simulink model "foc"  (R2026a)
settings: Solver=VariableStepAuto  FixedStep=5e-5
libraries: mcbcontrolslib x1, mcbplantlib x1, autolibpmsmexterior x1
settings Model: Creator=probst  LastModifiedBy=probst

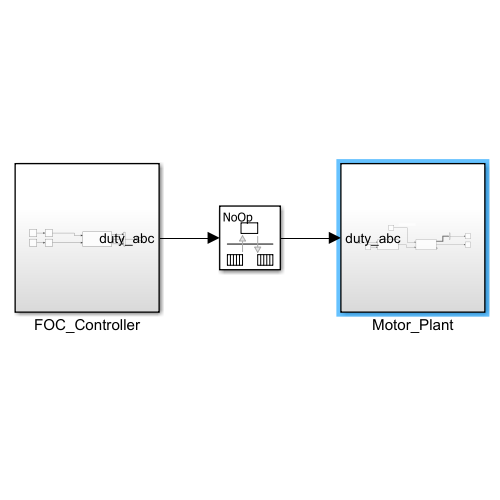
[thumbnail: Simulink's stored preview of the top-level diagram]
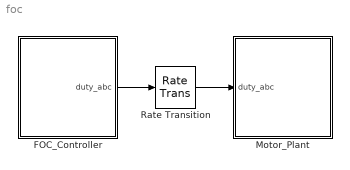
== system foc ==
  FOC_Controller : Subsystem
  Motor_Plant : Subsystem
  Rate Transition : RateTransition
  wires:
  FOC_Controller/1(duty_abc) -> Rate Transition/1
  Rate Transition/1 -> Motor_Plant/1(duty_abc)

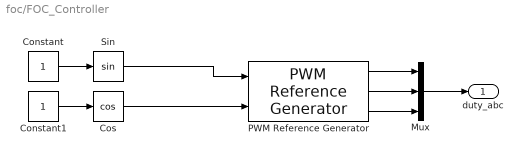
== system foc/FOC_Controller ==
  Constant : Constant
  Constant1 : Constant
  Cos : Trigonometry  Operator=cos
  Mux : Mux  Inputs=3
  PWM Reference Generator : mcbcontrolslib/PWM Reference Generator  modType=SVM: space vector modulation  inSignal=Valphabeta  expandVoltageInput=on  inputUnits=Per-unit  LimitModulation=off  enableVoltage=on  enableModulationSignal=off  enableDutyCycle=off  expandVoltageOutput=on
      settings: LibrarySourceBlock=mcblib/Controls/Math Transforms/PWM Reference Generator
  Sin : Trigonometry  OutputSignalType=real
  duty_abc : Outport
  wires:
  PWM Reference Generator/2 -> Mux/2
  PWM Reference Generator/1 -> Mux/1
  PWM Reference Generator/3 -> Mux/3
  Mux/1 -> duty_abc/1
  Sin/1 -> PWM Reference Generator/1
  Cos/1 -> PWM Reference Generator/2
  Constant/1 -> Sin/1
  Constant1/1 -> Cos/1

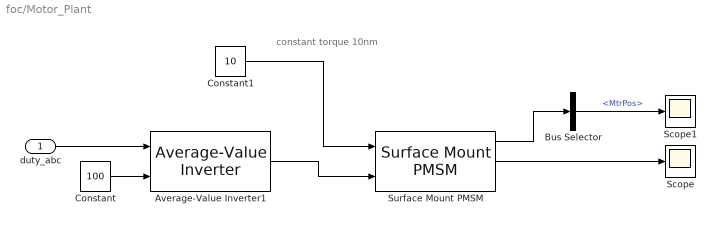
== system foc/Motor_Plant ==
  note: constant torque 10nm
  duty_abc : Inport
  Average-Value Inverter1 : mcbplantlib/Average-Value Inverter
      settings: LibrarySourceBlock=mcblib/Electrical Systems/Inverters/Average-Value Inverter
  Bus Selector : BusSelector  OutputSignals=MtrPos
  Constant : Constant  Value=100
  Constant1 : Constant  Value=10
  Scope : Scope
      settings: ActiveDisplayYMinimum=-2578.6954953565491  ActiveDisplayYMaximum=3666.8632765006746
  Scope1 : Scope
      settings: ActiveDisplayYMinimum=0.013250147681830247  ActiveDisplayYMaximum=0.022194753703218672
  Surface Mount PMSM : autolibpmsmexterior/Surface Mount PMSM  port_config=Torque  sim_type=Continuous  Ts=0.001  P=4  Rs=0.02  Ldq_=1.7e-3  KConstText=Permanent flux linkage constant (lambda_pm):  lambda_pm=0.2205  Ke=159.9771  Kt=1.323  mechanical=[0.0027, 4.924e-4, 0]  idq0=[0 0]  theta_init=0  omega_init=0  KConst=0.2205  lambda_pm_calc=0.2205  RefBlkName='autolibpmsmexterior/Surface Mount PMSM'  aMode=5  Ldq="[0.0017      0.0017]"
  wires:
  Average-Value Inverter1/1 -> Surface Mount PMSM/2
  Constant/1 -> Average-Value Inverter1/2
  duty_abc/1 -> Average-Value Inverter1/1
  Constant1/1 -> Surface Mount PMSM/1
  Surface Mount PMSM/2 -> Scope/1
  Surface Mount PMSM/1 -> Bus Selector/1
  Bus Selector/1 -> Scope1/1  "<MtrPos>"
